simulink model "Fix_out"  (R2022b)
settings: Solver=VariableStepAuto  StartTime=0.0  StopTime=10.0  RelTol=1e-3
settings Model: Creator=Km  LastModifiedBy=Km

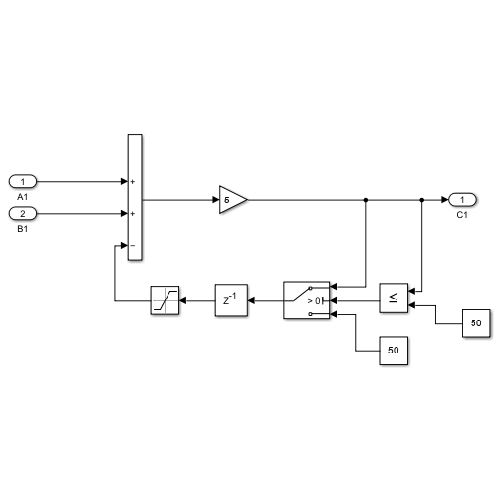
[thumbnail: Simulink's stored preview of the top-level diagram]
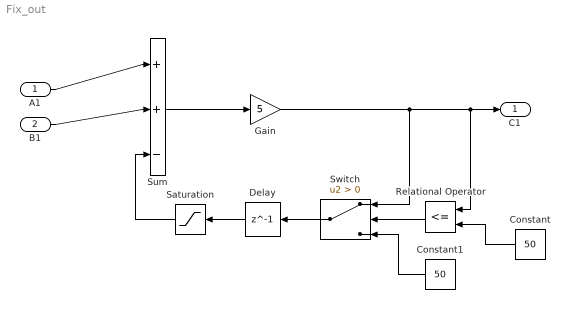
== system Fix_out ==
  A1 : Inport
  B1 : Inport  Port=2
  Constant : Constant  Value=50
  Constant1 : Constant  Value=50
  Delay : Delay  DelayLength=1  InitialCondition=0
  Gain : Gain  Gain=5
  Relational Operator : RelationalOperator  Operator=<=  OutDataTypeStr=boolean  RndMeth=Simplest  InputSameDT=off
  Saturation : Saturate  UpperLimit=100  LowerLimit=-100
  Sum : Sum  Inputs=|++-
  Switch : Switch  Criteria=u2 > Threshold  SaturateOnIntegerOverflow=off  InputSameDT=off
  C1 : Outport
  wires:
  Constant1/1 -> Switch/3
  Relational Operator/1 -> Switch/2
  Constant/1 -> Relational Operator/2
  Switch/1 -> Delay/1
  A1/1 -> Sum/1
  B1/1 -> Sum/2
  Sum/1 -> Gain/1
  Delay/1 -> Saturation/1
  Saturation/1 -> Sum/3
  Gain/1 -> Switch/1, Relational Operator/1, C1/1
